simulink model "Missile_C_Y"  (R2018b)
settings: Solver=ode4  StartTime=0.0  StopTime=5  FixedStep=Step_Size  RelTol=1e-3  EnableMultiTasking=on
InitFcn:
  | clc ;
  | clear all ;
  | close all ;
  | Missile_Data ;
  | Sim_Parameters ;
undefined symbols (not defined in the file): Tbl_ALPHAT, Tbl_CY_DEL_Y, Tbl_CY_PHIT, Tbl_MACH
libraries: simulink_extras x2
settings Model: Creator=e803534  LastModifiedBy=auten
settings OptimizationCC: LifeSpan=inf
settings DebuggingCC: UnconnectedInputMsg=none  UnconnectedOutputMsg=none  UnconnectedLineMsg=none  SFUnexpectedBacktrackingDiag=warning  SFNoUnconditionalDefaultTransitionDiag=warning
settings SFSimCC: SimUseLocalCustomCode=off
settings RTWCC: RTWUseLocalCustomCode=off
settings CodeAppCC: StateflowObjectComments=on
settings GRTTargetCC: TargetLangStandard=C89/C90 (ANSI)  GeneratePreprocessorConditionals=Disable all
settings ConfigComp: CovMetricSettings=dw  CovHtmlReporting=on  CovSaveCumulativeToWorkspaceVar=on  CovSaveSingleToWorkspaceVar=on  CovExternalEMLEnable=off

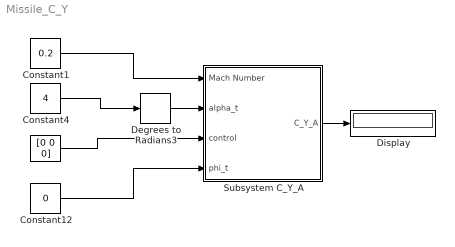
== system Missile_C_Y ==
  " " : Constant  Value=[0 0 0]  VectorParams1D=off  SampleTime=-1
  Constant1 : Constant  Value=0.2
  Constant12 : Constant  Value=0
  Constant4 : Constant  Value=4
  Degrees to Radians3 : simulink_extras/Transformations/Degrees to Radians
  Display : Display
  Subsystem C_Y_A : Subsystem
  wires:
  Constant1/1 -> Subsystem C_Y_A/1(Mach Number)
  Constant4/1 -> Degrees to Radians3/1
  Subsystem C_Y_A/1(C_Y_A) -> Display/1
  Constant12/1 -> Subsystem C_Y_A/4(phi_t)
  Degrees to Radians3/1 -> Subsystem C_Y_A/2(alpha_t)
  " "/1 -> Subsystem C_Y_A/3(control)

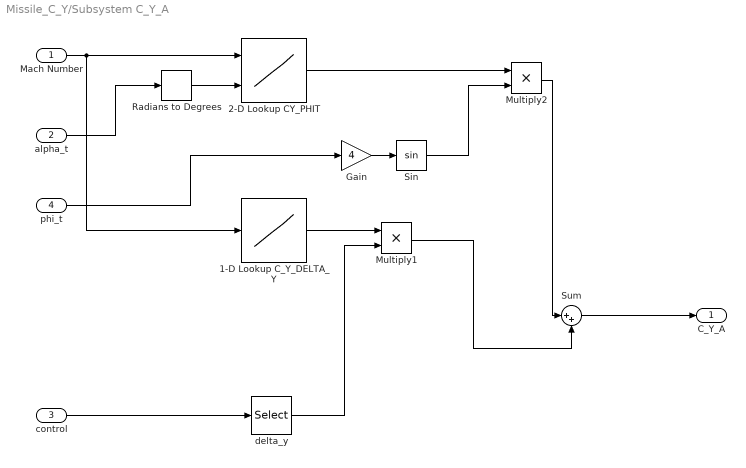
== system Missile_C_Y/Subsystem C_Y_A ==
  Mach Number : Inport
  alpha_t : Inport  Port=2
  control : Inport  Port=3
  phi_t : Inport  Port=4
  1-D Lookup C_Y_DELTA_Y : Lookup_n-D  NumberOfTableDimensions=1  BreakpointsForDimension1=Tbl_MACH  Table=Tbl_CY_DEL_Y  InternalRulePriority=Speed  RndMeth=Simplest  InputSameDT=on
  2-D Lookup CY_PHIT : Lookup_n-D  BreakpointsForDimension1=Tbl_MACH  BreakpointsForDimension2=Tbl_ALPHAT  Table=Tbl_CY_PHIT  InternalRulePriority=Speed  RndMeth=Simplest  InputSameDT=on
  Gain : Gain  Gain=4
  Multiply1 : Product
  Multiply2 : Product
  Radians to Degrees : simulink_extras/Transformations/Radians to Degrees
  Sin : Trigonometry
  Sum : Sum  Inputs=|++
  delta_y : Selector  InputPortWidth=3  IndexOptions=Index vector (dialog)  Indices=[3]  OutputSizes=1
  C_Y_A : Outport
  wires:
  Multiply1/1 -> Sum/2
  1-D Lookup C_Y_DELTA_Y/1 -> Multiply1/1
  2-D Lookup CY_PHIT/1 -> Multiply2/1
  Mach Number/1 -> 1-D Lookup C_Y_DELTA_Y/1, 2-D Lookup CY_PHIT/1
  Sum/1 -> C_Y_A/1
  Gain/1 -> Sin/1
  phi_t/1 -> Gain/1
  control/1 -> delta_y/1
  alpha_t/1 -> Radians to Degrees/1
  delta_y/1 -> Multiply1/2
  Sin/1 -> Multiply2/2
  Multiply2/1 -> Sum/1
  Radians to Degrees/1 -> 2-D Lookup CY_PHIT/2
